simulink model "lqr_verify"  (R2024b)
settings: Solver=FixedStepDiscrete  StartTime=0.0  StopTime=10.0  FixedStep=0.001  RelTol=1e-3
values from neighbouring files (symbols this model uses):
  Ad = sys_d.A    [calc_lqr.m]
  Bd = sys_d.B    [calc_lqr.m]
  K = 0.000004057    (= 4.057e-06)    [calc_lqr.m]
  Ts = 0.001    [calc_lqr.m]
undefined symbols (not defined in the file or in its folder): DiscIntNeverNeededParam
settings Model: Creator=yangchaojie  LastModifiedBy=yangchaojie

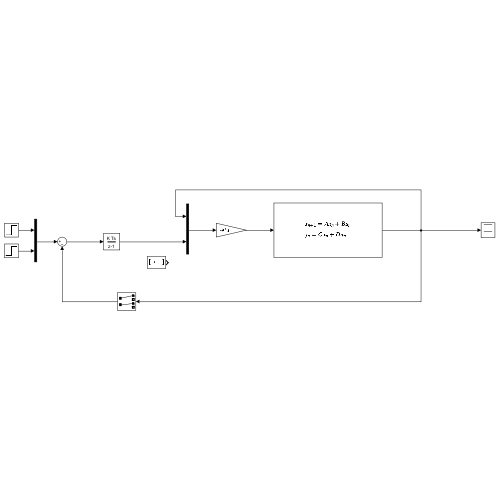
[thumbnail: Simulink's stored preview of the top-level diagram]
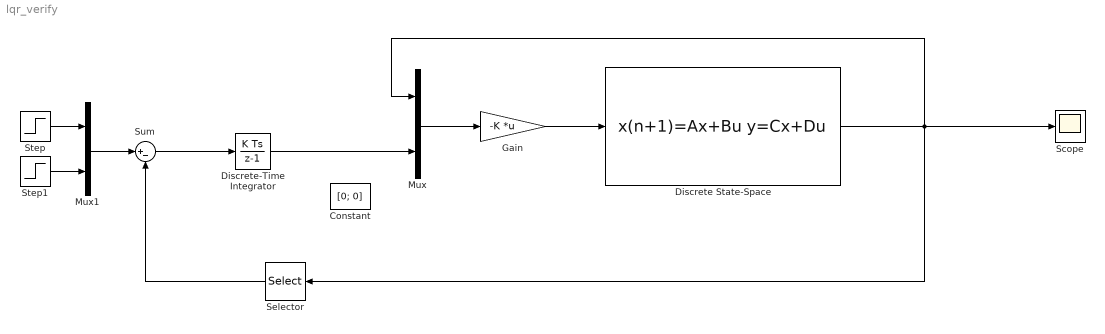
== system lqr_verify ==
  Constant : Constant  Value=[0; 0]
  Discrete State-Space : DiscreteStateSpace  A=Ad  B=Bd  C=eye(4)  D=zeros(4,2)  InitialCondition=[0; 0; 0; 0.1]  SampleTime=Ts
  Discrete-Time Integrator : DiscreteIntegrator  SampleTime=Ts  ICPrevOutput=DiscIntNeverNeededParam  ICPrevScaledInput=DiscIntNeverNeededParam
  Gain : Gain  Gain=-K  Multiplication=Matrix(K*u)
  Mux : Mux  Inputs=2
  Mux1 : Mux  Inputs=2
  Scope : Scope
  Selector : Selector  InputPortWidth=4  IndexOptions=Index vector (dialog)  Indices=[1 3]  OutputSizes=1
  Step : Step  SampleTime=Ts
  Step1 : Step  SampleTime=Ts
  Sum : Sum  Inputs=|+-
  wires:
  Discrete State-Space/1 -> Selector/1, Mux/1, Scope/1
  Selector/1 -> Sum/2
  Mux/1 -> Gain/1
  Gain/1 -> Discrete State-Space/1
  Sum/1 -> Discrete-Time Integrator/1
  Step/1 -> Mux1/1
  Step1/1 -> Mux1/2
  Mux1/1 -> Sum/1
  Discrete-Time Integrator/1 -> Mux/2
